simulink model "sus_veh_"  (R2018b)
settings: Solver=VariableStepAuto  StartTime=0.0  StopTime=60  RelTol=1e-3
undefined symbols (not defined in the file): b, k1, k2, m1, m2
settings Model: Creator=Acer  LastModifiedBy=Acer
settings DataIOCC: ReturnWorkspaceOutputs=on

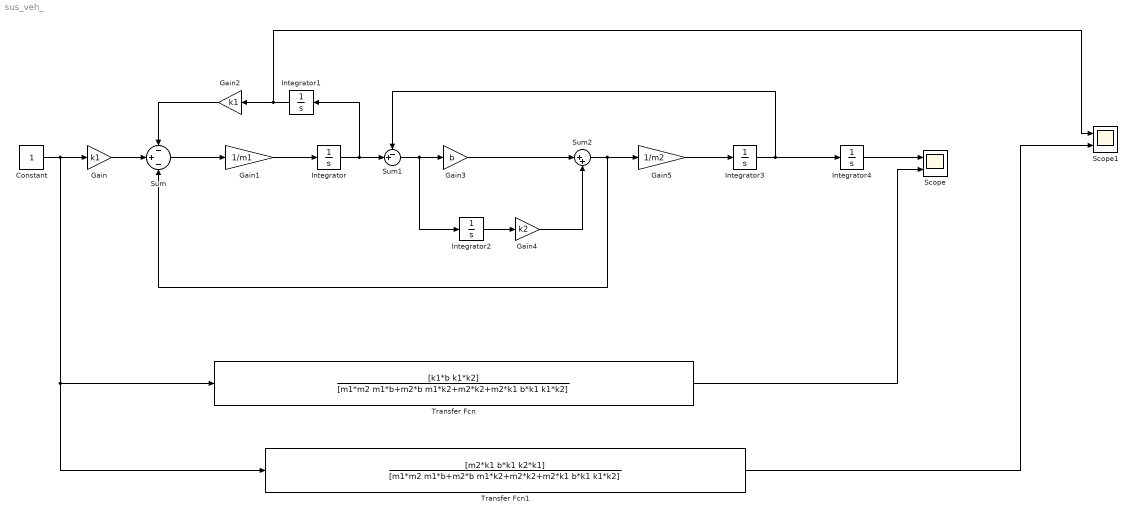
== system sus_veh_ ==
  Constant : Constant
  Gain : Gain  Gain=k1
  Gain1 : Gain  Gain=1/m1
  Gain2 : Gain  Gain=k1
  Gain3 : Gain  Gain=b
  Gain4 : Gain  Gain=k2
  Gain5 : Gain  Gain=1/m2
  Integrator{,1..4} (5 alike) : Integrator
  Scope : Scope  NumInputPorts=2
  Scope1 : Scope  NumInputPorts=2
  Sum : Sum  Inputs=-+-
  Sum1 : Sum  Inputs=-+|
  Sum2 : Sum  Inputs=|++
  Transfer Fcn : TransferFcn  Numerator=[k1*b k1*k2]  Denominator=[m1*m2 m1*b+m2*b m1*k2+m2*k2+m2*k1 b*k1 k1*k2]
  Transfer Fcn1 : TransferFcn  Numerator=[m2*k1 b*k1 k2*k1]  Denominator=[m1*m2 m1*b+m2*b m1*k2+m2*k2+m2*k1 b*k1 k1*k2]
  wires:
  Gain/1 -> Sum/2
  Constant/1 -> Transfer Fcn1/1, Transfer Fcn/1, Gain/1
  Sum/1 -> Gain1/1
  Gain1/1 -> Integrator/1
  Gain2/1 -> Sum/1
  Integrator/1 -> Sum1/2, Integrator1/1
  Sum1/1 -> Integrator2/1, Gain3/1
  Integrator2/1 -> Gain4/1
  Gain3/1 -> Sum2/1
  Gain4/1 -> Sum2/2
  Sum2/1 -> Sum/3, Gain5/1
  Gain5/1 -> Integrator3/1
  Integrator3/1 -> Integrator4/1, Sum1/1
  Integrator4/1 -> Scope/1
  Transfer Fcn/1 -> Scope/2
  Integrator1/1 -> Gain2/1, Scope1/1
  Transfer Fcn1/1 -> Scope1/2
